simulink model "blind_cop"  (Simulink 8.7)
settings: Solver=FixedStepAuto  StartTime=0.0  StopTime=10.0  FixedStep=0.01  RelTol=1e-3
settings Model: Creator=eispin  LastModifiedBy=eispin
settings DataIOCC: LimitDataPoints=off  SaveFormat=Dataset
settings DebuggingCC: UnderspecifiedInitializationDetection=Simplified  MergeDetectMultiDrivingBlocksExec=error
settings HardwareCC: ProdBitPerPointer=64  ProdLargestAtomicFloat=Float  ProdIntDivRoundTo=Zero  ProdEndianess=LittleEndian  ProdWordSize=64  ProdHWDeviceType=Intel->x86-64 (Windows64)
settings ModelReferenceCC: PropagateSignalLabelsOutOfModel=on
settings ConfigComp: CovModelRefEnable=off

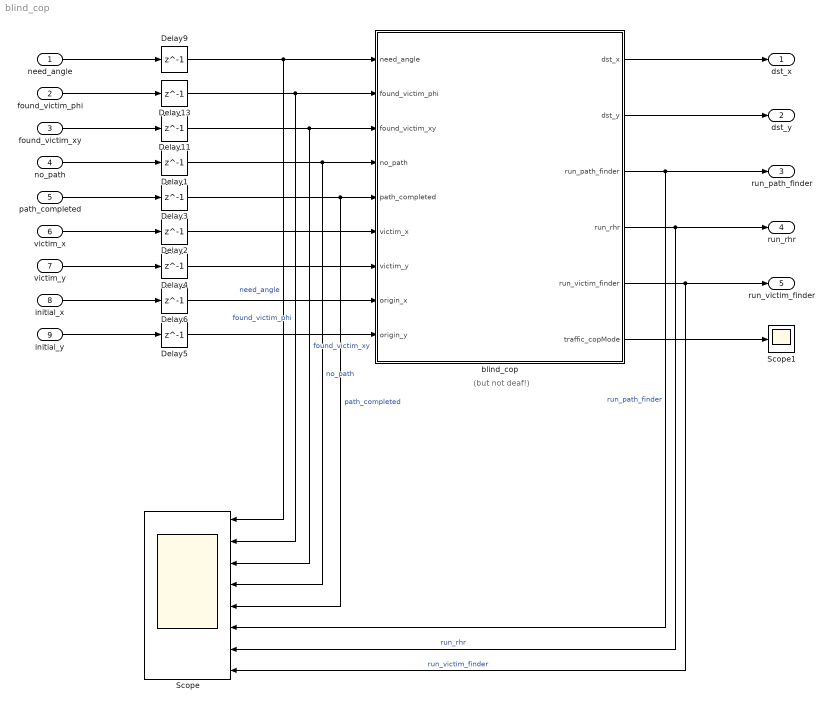
== system blind_cop ==
  note: (but not deaf!)
  need_angle : Inport
  found_victim_phi : Inport  Port=2
  found_victim_xy : Inport  Port=3
  no_path : Inport  Port=4
  path_completed : Inport  Port=5
  victim_x : Inport  Port=6
  victim_y : Inport  Port=7
  initial_x : Inport  Port=8
  initial_y : Inport  Port=9
  Delay{1..6,9,11,13} (9 alike) : Delay  DelayLength=1
  Scope : Scope  NumInputPorts=8
  Scope1 : Scope
  blind_cop : Stateflow chart  TreatAsAtomicUnit=on
  dst_x : Outport
  dst_y : Outport  Port=2
  run_path_finder : Outport  Port=3
  run_rhr : Outport  Port=4
  run_victim_finder : Outport  Port=5
  wires:
  blind_cop/5(run_victim_finder) -> Scope/8, run_victim_finder/1  "run_victim_finder"
  blind_cop/3(run_path_finder) -> Scope/6, run_path_finder/1  "run_path_finder"
  blind_cop/4(run_rhr) -> Scope/7, run_rhr/1  "run_rhr"
  blind_cop/2(dst_y) -> dst_y/1
  blind_cop/1(dst_x) -> dst_x/1
  blind_cop/6(traffic_copMode) -> Scope1/1
  found_victim_xy/1 -> Delay11/1
  no_path/1 -> Delay1/1
  found_victim_phi/1 -> Delay13/1
  initial_y/1 -> Delay5/1
  victim_y/1 -> Delay4/1
  victim_x/1 -> Delay2/1
  path_completed/1 -> Delay3/1
  initial_x/1 -> Delay6/1
  need_angle/1 -> Delay9/1
  Delay11/1 -> Scope/3, blind_cop/3(found_victim_xy)  "found_victim_xy"
  Delay6/1 -> blind_cop/8(origin_x)
  Delay4/1 -> blind_cop/7(victim_y)
  Delay9/1 -> Scope/1, blind_cop/1(need_angle)  "need_angle"
  Delay13/1 -> Scope/2, blind_cop/2(found_victim_phi)  "found_victim_phi"
  Delay5/1 -> blind_cop/9(origin_y)
  Delay3/1 -> Scope/5, blind_cop/5(path_completed)  "path_completed"
  Delay1/1 -> Scope/4, blind_cop/4(no_path)  "no_path"
  Delay2/1 -> blind_cop/6(victim_x)

== stateflow chart blind_cop ==
  state GetTheLadiesOrGentlemen
    % Done ^.^
    entry:
    run_path_finder = 0;
  state NoPathFound
    % fault tolerance state: no path found but
    % by assumtions there is one -> faulty sensor data -> RHR
    entry:
    run_rhr = 1;
    run_path_finder = 0;
    exit:
    run_rhr = 0;
  state FollowPath
    state RunToVictim
      entry:
      run_rhr = 0;
      run_path_finder = 1;
      run_victim_finder = 0;
      dst_x = victim_x;
      dst_y = victim_y;
    state GetOuttaHere
      entry:
      run_path_finder = 1;
      dst_x = origin_x;
      dst_y = origin_y;
    state Docking
      % no-op
    state WaitPathZero
      entry:
      run_path_finder = 0;
    (default) -> RunToVictim
    RunToVictim -> WaitPathZero : [path_completed == 1]
    WaitPathZero -> Docking : [path_completed == 0]
    Docking -> GetOuttaHere : [after(0.1, sec)]
  state InitialRHR
    state InitialRHR
      entry:
      run_rhr = 1;
      run_path_finder = 0;
      run_victim_finder = 0;
    state SenseAngle
      entry:
      run_rhr = 0;
      run_victim_finder = 1;
    state WaitAngleZero
      entry:
      run_victim_finder = 0;
    (default) -> InitialRHR.InitialRHR
    InitialRHR.InitialRHR -> SenseAngle : [need_angle == 1]
    SenseAngle -> WaitAngleZero : [found_victim_phi == 1]
    WaitAngleZero -> InitialRHR.InitialRHR : [found_victim_phi == 0]
  (default) -> InitialRHR
  InitialRHR -> FollowPath : [found_victim_xy == 1]
  FollowPath -> NoPathFound : [no_path == 1]
  NoPathFound -> (history) : [after(30, sec)]
  GetOuttaHere -> GetTheLadiesOrGentlemen : [path_completed == 1]
  data: need_angle input double; found_victim_phi input double; found_victim_xy input double; no_path input double; path_completed input double; victim_x input double; victim_y input double; origin_x input double; origin_y input double; dst_x output double; dst_y output double; run_path_finder output double =0; run_rhr output double =0; run_victim_finder output double =0; traffic_copMode output Enum: traffic_copModeType3; last_x local double; last_y local double; far_enough local double; enable_first_scan local double
